simulink model "RBNN_NNT_timing_of_learning_1layerRBNN32order"  (R2019a)
settings: Solver=FixedStepAuto  StartTime=0.0  StopTime=inf  FixedStep=0.000001  RelTol=1e-3
libraries: dspstat3 x6, dspxfrm3 x1
(part 1 of 3)
settings Model: NumberOfSteps=3200  Creator=vardhah  LastModifiedBy=vardhah
settings DataIOCC: ReturnWorkspaceOutputs=off
settings DebuggingCC: UnderSpecifiedDimensionMsg=warning  ArithmeticOperatorsInVariantConditions=warning

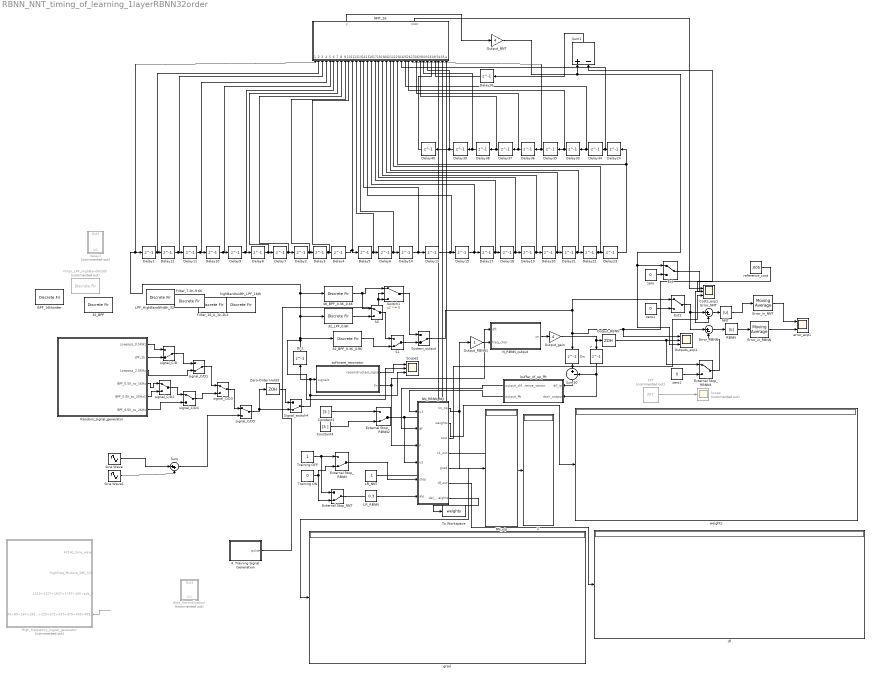
== system RBNN_NNT_timing_of_learning_1layerRBNN32order ==
  32_BPF : DiscreteFir  Tag=BlockMethodSubSystem  Coefficients=[0.0231270967292107159 0.0175343355945324977 0.00605221670125152041 0 0.00719679767045157404 0.0248456434051700405 0.0392205491332038511 0.0335684455675286375 -2.98876364449908766e-17 -0.0522852296501915767 -0.0987039819924426381 -0.111406686169706906 -0.0755372385277077452 1.2744675147390013e-17 0.0844207978699620387 0.139588301189413205 0.139588301189413205 0.0844207978699620387 1.2744675147390013e-17 -0.0755372385277077452 -0.111406686169706906 -0.0987039819924426381 -0.0522852296501915767 -2.98876364449908766e-17 0.0335684455675286375 0.0392205491332038511 0.0248456434051700405 0.00719679767045157404 0 0.00605221670125152041 0.0175343355945324977 0.0231270967292107159]  InputProcessing=Columns as channels (frame based)
  32_BPF_0.3K_0.9K : DiscreteFir  Tag=BlockMethodSubSystem  Coefficients=[0.00662659845422776134 0.00983298588902027475 0.00809664409693275702 -5.79647672595923754e-18 -0.0141669692502708264 -0.0321973902262055467 -0.0502752481995635894 -0.0637677476357453449 -0.0683320878931848175 -0.0610667384383032988 -0.0414056635152443217 -0.0115027859073064606 0.0240263013390189448 0.0589774451458855986 0.0868579066741778927 0.102309229147061892 0.102309229147061892 0.0868579066741778927 0.0589774451458855986 0.0240263013390189448 -0.0115027859073064606 -0.0414056635152443217 -0.0610667384383032988 -0.0683320878931848175 -0.0637677476357453449 -0.0502752481995635894 -0.0321973902262055467 -0.0141669692502708264 -5.79647672595923754e-18 0.00809664409693275702 0.00983298588902027475 0.00662659845422776134]  InputProcessing=Columns as channels (frame based)  SampleTime=0.0001
  32_LPF_0.6K : DiscreteFir  Tag=BlockMethodSubSystem  Coefficients=[-0.00901248685369954346 -0.0166232313070880447 -0.02293849257176446 -0.0268238277900753851 -0.0272765662653831481 -0.0235546351369226477 -0.0152840059258895229 -0.00253072016398011397 0.0141728632030948976 0.0338528489286080425 0.055168937477022735 0.0765332041207810732 0.0962604488743150494 0.112734006746784729 0.124568738621398098 0.130752918042798372 0.130752918042798372 0.124568738621398098 0.112734006746784729 0.0962604488743150494 0.0765332041207810732 0.055168937477022735 0.0338528489286080425 0.0141728632030948976 -0.00253072016398011397 -0.0152840059258895229 -0.0235546351369226477 -0.0272765662653831481 -0.0268238277900753851 -0.02293849257176446 -0.0166232313070880447 -0.00901248685369954346]  InputProcessing=Columns as channels (frame based)  SampleTime=0.0001
  4. Training Signal Generation : MATLAB Function  TreatAsAtomicUnit=on
  48_BPF_0.3K_0.6K : DiscreteFir  Tag=BlockMethodSubSystem  Coefficients=[0.0173870629140374378 0.0207423482676672884 0.0225684944558904275 0.0223574555139875765 0.0197817601251017959 0.0147549785512151154 0.00746744065508679611 -0.001608996203153008 -0.0117498180199336073 -0.0220390277764995618 -0.0314572377427717528 -0.0389877339734026607 -0.0437289550833909607 -0.0450005271887067293 -0.0424302142891804998 -0.0360109004456410225 -0.0261198472327749086 -0.0134966227084623806 0.00081920313306374482 0.0155848141621206405 0.0294754638356683092 0.0412174342630990259 0.0497181612101459114 0.0541791579705657028 0.0541791579705657028 0.0497181612101459114 0.0412174342630990259 0.0294754638356683092 0.0155848141621206405 0.00081920313306374482 -0.0134966227084623806 -0.0261198472327749086 -0.0360109004456410225 -0.0424302142891804998 -0.0450005271887067293 -0.0437289550833909607 -0.0389877339734026607 -0.0314572377427717528 -0.0220390277764995618 -0.0117498180199336073 -0.001608996203153008 0.00746744065508679611 0.0147549785512151154 0.0197817601251017959 0.0223574555139875765 0.0225684944558904275 0.0207423482676672884 0.0173870629140374378]  InputProcessing=Columns as channels (frame based)  SampleTime=0.0001
  BPF_16thorder : DiscreteFir  Tag=BlockMethodSubSystem  Coefficients=[-0.0560788660629819163 -0.080220031928137342 -0.085169812197034192 -0.0616477005407154097 -0.0104987832754634518 0.0560691321297696263 0.118166811935027122 0.155549755804414214 0.155549755804414214 0.118166811935027122 0.0560691321297696263 -0.0104987832754634518 -0.0616477005407154097 -0.085169812197034192 -0.080220031928137342 -0.0560788660629819163]  InputProcessing=Columns as channels (frame based)  SampleTime=0.0001
  Constant1 : Constant  Value=[5 ]
  Constant4 : Constant  Value=[3 ]
  Costs_exp1 : Scope  NumInputPorts=3
  Delay{1..24,33..40} (32 alike) : Delay  DelayLength=1  InitialCondition=0
  Dn : Delay  DelayLength=1  InitialCondition=0
  Dn1 : Delay  DelayLength=1  InitialCondition=0
  Error_NNT : Sum  Inputs=|+-
  Error_RBNN : Sum  Inputs=|+-
  Error_in_NNT : dspstat3/Moving Average  Method=Sliding window  ForgettingFactorPort=off  SpecifyWindowLength=on  WindowLength=32  ForgettingFactor=0.9  SimulateUsing=Code generation
  Error_in_RBNN : dspstat3/Moving Average  Method=Sliding window  ForgettingFactorPort=off  SpecifyWindowLength=on  WindowLength=32  ForgettingFactor=0.9  SimulateUsing=Code generation
  Ext : ManualSwitch
  Ext1 : ManualSwitch
  External Stop_NNT : ManualSwitch  CurrentSetting=0
  External Stop_RBNN : ManualSwitch  CurrentSetting=0
  External Stop_RBNN2 : ManualSwitch  CurrentSetting=0
  External Stop_RBNN3 : ManualSwitch
  FFT : dspxfrm3/FFT  Commented=on  FFTImplementation=Auto  CompMethod=Table lookup  TableOpt=NEW  TableOptActive=Speed  BitRevOrder=off  Normalize=off  InheritFFTLength=off  FFTLength=16  WrapInput=on  roundingMode=Floor  overflowMode=off  firstCoeffDataTypeStr=Inherit: Same word length as input  firstCoeffLastDataTypeStr=Inherit: Same word length as input  outputMin=[]  outputMax=[]
  Filter_16_A_1k-2k2 : DiscreteFir  Tag=BlockMethodSubSystem  Coefficients=[-0.198889914644374777 0.0882189428518377339 0.0736891495871065116 0.0638368801789635787 0.0566372642221577294 0.0523172683654103132 0.0494565343907736044 0.048157521822162791 0.048157521822162791 0.0494565343907736044 0.0523172683654103132 0.0566372642221577294 0.0638368801789635787 0.0736891495871065116 0.0882189428518377339 -0.198889914644374777]  InputProcessing=Columns as channels (frame based)  SampleTime=0.0001
  "Filter_7.2K-9.6K " : DiscreteFir  Tag=BlockMethodSubSystem  Coefficients=[-0.0120785049852322399 -0.0942455273574688279 0.0101245004695954266 0.125460404555770566 0.034165372769331126 -0.1614987160724079 -0.0984930555982914957 0.150982315564688691 0.150982315564688691 -0.0984930555982914957 -0.1614987160724079 0.034165372769331126 0.125460404555770566 0.0101245004695954266 -0.0942455273574688279 -0.0120785049852322399]  InputProcessing=Columns as channels (frame based)  SampleTime=0.0001
  Filter_LPF_HighBandWidth : DiscreteFir  Tag=BlockMethodSubSystem  Commented=on  Coefficients=[0.00257561197553052117 0.0149226993015543988 -0.0126813197622564593 0.0131583623867790739 -0.0109438145213804211 0.00462377218068549256 0.00574880781840408916 -0.0188595701191665473 0.032156879848246514 -0.042054633169390801 0.0443249918452583783 -0.0343435917303160365 0.00670297923827019304 0.0478068572768818173 -0.160206703181909604 0.618531838092966302 0.618531838092966302 -0.160206703181909604 0.0478068572768818173 0.00670297923827019304 -0.0343435917303160365 0.0443249918452583783 -0.042054633169390801 0.032156879848246514 -0.0188595701191665473 0.00574880781840408916 0.00462377218068549256 -0.0109438145213804211 0.0131583623867790739 -0.0126813197622564593 0.0149226993015543988 0.00257561197553052117]  InputProcessing=Columns as channels (frame based)  SampleTime=0.0001
  HIgh_frequency_signal_generator : Subsystem  Commented=on
  LPF_HighBandWidth_32 : DiscreteFir  Tag=BlockMethodSubSystem  Coefficients=[0.00257561197553052117 0.0149226993015543988 -0.0126813197622564593 0.0131583623867790739 -0.0109438145213804211 0.00462377218068549256 0.00574880781840408916 -0.0188595701191665473 0.032156879848246514 -0.042054633169390801 0.0443249918452583783 -0.0343435917303160365 0.00670297923827019304 0.0478068572768818173 -0.160206703181909604 0.618531838092966302 0.618531838092966302 -0.160206703181909604 0.0478068572768818173 0.00670297923827019304 -0.0343435917303160365 0.0443249918452583783 -0.042054633169390801 0.032156879848246514 -0.0188595701191665473 0.00574880781840408916 0.00462377218068549256 -0.0109438145213804211 0.0131583623867790739 -0.0126813197622564593 0.0149226993015543988 0.00257561197553052117]  InputProcessing=Columns as channels (frame based)  SampleTime=0.0001
  LR_NNT : Constant  Value=.1
  LR_RBNN : Constant  Value=0.3
  NNT : Abs
  NNT_16 : MATLAB Function  TreatAsAtomicUnit=on  SystemSampleTime=0.0001
  NN_RBNN_NN : MATLAB Function  TreatAsAtomicUnit=on
  NN_o/p : Display
  N_RBNN_output : MATLAB Function  TreatAsAtomicUnit=on
  Output_NNT : Gain  Gain=4
  Output_RBNN : ZeroOrderHold  SampleTime=-1
  Output_RBNN1 : Gain
  Output_gain : Gain  Gain=4
  Outputs_exp1 : Scope  NumInputPorts=3
  RBNN : Abs
  Random_signal_generator : Subsystem
  S1 : ManualSwitch  CurrentSetting=0
  S3 : ManualSwitch
  Scope : Scope  Commented=on
  Scope2 : Scope  NumInputPorts=3
  Signal_switch4 : ManualSwitch  CurrentSetting=0
  Sine Wave : Sin  Frequency=1297  SampleTime=0.0001
  Sine Wave1 : Sin  Frequency=2031  SampleTime=0.0001
  Sum : Sum  Inputs=|++
  Sum1 : Sum  Inputs=+-
  Sum50 : Sum  Inputs=|+-
  Switch1 : Switch  Criteria=u2 ~= 0
  "System_output " : ManualSwitch  CurrentSetting=0
  To Workspace : ToWorkspace  VariableName=weights  SaveFormat=Timeseries  SampleTime=-1
  Training OFF : Constant
  Training ON : Constant  Value=0
  Z : Display
  Zero-Order Hold3 : ZeroOrderHold  SampleTime=0.0001
  buffer_of_op_fft : MATLAB Function  TreatAsAtomicUnit=on
  data_Normalization : Subsystem  Commented=on
  delay1 : Subsystem  Commented=on
  df : Display
  error_exp1 : Scope  NumInputPorts=2
  grad : Display
  highBandwidth_LPF_16th : DiscreteFir  Tag=BlockMethodSubSystem  Coefficients=[-0.0297618438739734592 -0.0348768570143923456 0.0417652636536197108 0.0516071256815222451 -0.0669316025800295866 -0.0943151588376726635 0.157872597041064711 0.474640475929861472 0.474640475929861472 0.157872597041064711 -0.0943151588376726635 -0.0669316025800295866 0.0516071256815222451 0.0417652636536197108 -0.0348768570143923456 -0.0297618438739734592]  InputProcessing=Columns as channels (frame based)  SampleTime=0.0001
  reference_cost : Constant  Value=.005
  signal_C/D : ManualSwitch  CurrentSetting=0
  signal_C/D1 : ManualSwitch  CurrentSetting=0
  signal_C/D{2..5} (4 alike) : ManualSwitch
  software_rezonator : MATLAB Function  TreatAsAtomicUnit=on  SystemSampleTime=0.0001
  weights : Display
  y : Delay  DelayLength=1  InitialCondition=0
  zero : Constant  Value=0
  zero1 : Constant  Value=0
  "zero1 " : Constant  Value=0
  wires:
  software_rezonator/1(reconstructed_signal) -> Scope2/1
  software_rezonator/2(Fn) -> NN_RBNN_NN/3(F), N_RBNN_output/1(dft)
  N_RBNN_output/1(yn) -> Output_gain/1
  Dn/1 -> Sum50/1
  y/1 -> buffer_of_op_fft/2(rbnn_output), Sum50/2
  NN_RBNN_NN/1(nn_op) -> NN_o/p/1, Output_RBNN1/1
  Training OFF/1 -> External Stop_NNT/1, External Stop_RBNN/1
  Training ON/1 -> External Stop_NNT/2, External Stop_RBNN/2
  NN_RBNN_NN/3(cost) -> Costs_exp1/3
  NN_RBNN_NN/2(weights) -> weights/1
  NN_RBNN_NN/4(z1_out) -> Z/1
  Sum50/1 -> buffer_of_op_fft/1(dif_ip)
  buffer_of_op_fft/1(output_difference_vector) -> NN_RBNN_NN/2(df)
  buffer_of_op_fft/2(output_fft) -> NN_RBNN_NN/1(u1)
  NNT_16/1(y) -> Output_NNT/1
  Delay16/1 -> NNT_16/33(df)
  Delay4/1 -> NNT_16/11(X10), Delay5/1
  Delay6/1 -> Delay14/1, NNT_16/13(X12)
  Delay5/1 -> Delay6/1, NNT_16/12(X11)
  Delay2/1 -> Delay3/1, NNT_16/9(X8)
  Delay13/1 -> NNT_16/15(X14), Delay15/1
  Delay14/1 -> Delay13/1, NNT_16/14(X13)
  Delay10/1 -> NNT_16/5(X4), Delay9/1
  signal_C/D5/1 -> Zero-Order Hold3/1, Signal_switch4/2
  Delay3/1 -> NNT_16/10(X9), Delay4/1
  Delay7/1 -> Delay2/1, NNT_16/8(X7)
  Delay8/1 -> NNT_16/7(X6), Delay7/1
  Delay1/1 -> Delay12/1, NNT_16/2(X1)
  Delay9/1 -> NNT_16/6(X5), Delay8/1
  Delay12/1 -> NNT_16/3(X2), Delay11/1
  Delay11/1 -> NNT_16/4(X3), Delay10/1
  Sum1/1 -> Delay16/1
  Error_RBNN/1 -> RBNN/1
  Error_NNT/1 -> NNT/1
  LR_RBNN/1 -> NN_RBNN_NN/6(alp)
  RBNN/1 -> Error_in_RBNN/1
  NNT/1 -> Error_in_NNT/1
  Error_in_NNT/1 -> error_exp1/1
  Error_in_RBNN/1 -> error_exp1/2
  External Stop_NNT/1 -> NNT_16/34(stop)
  Output_gain/1 -> y/1, Output_RBNN/1
  LR_NNT/1 -> NNT_16/35(alpha_l)
  HIgh_frequency_signal_generator/4(43+89+167+193+229+271+337+379+409+499_H) -> ?
  Zero-Order Hold3/1 -> Signal_switch4/1
  FFT/1 -> Scope/1
  Switch1/1 -> "System_output "/1
  Constant1/1 -> External Stop_RBNN2/1
  4. Training Signal Generation/1(pulse) -> Switch1/3, Switch1/2
  Constant4/1 -> External Stop_RBNN2/2
  External Stop_RBNN2/1 -> NNT_16/36(a), NN_RBNN_NN/4(u2)
  Output_NNT/1 -> Outputs_exp1/3, Ext/1, Sum1/1
  S3/1 -> S1/1
  S1/1 -> "System_output "/2
  Output_RBNN1/1 -> N_RBNN_output/2(freq_char)
  NN_RBNN_NN/5(grad) -> grad/1
  Output_RBNN/1 -> External Stop_RBNN3/1, Outputs_exp1/2
  NN_RBNN_NN/6(df_out) -> df/1
  "System_output "/1 -> Ext1/1, Dn/1, Sum1/2, Outputs_exp1/1
  NN_RBNN_NN/7(del_weights) -> To Workspace/1
  Signal_switch4/1 -> Scope2/3, Dn1/1, software_rezonator/1(signalz)
  signal_C/D/1 -> signal_C/D1/1
  Random_signal_generator/3(Lowpass_2.5KHz) -> signal_C/D1/2
  Random_signal_generator/4(BPF_0.5K_to_1KHz) -> signal_C/D2/1
  signal_C/D3/1 -> signal_C/D5/1
  signal_C/D1/1 -> signal_C/D3/1
  Random_signal_generator/1(Lowpass_0.5KHz) -> signal_C/D/1
  Random_signal_generator/2(LPF_1k) -> signal_C/D/2
  "zero1 "/1 -> External Stop_RBNN3/2
  External Stop_RBNN3/1 -> Error_RBNN/2
  Ext/1 -> Error_NNT/2
  zero/1 -> Ext/2
  zero1/1 -> Ext1/2
  Ext1/1 -> Error_RBNN/1, Error_NNT/1
  reference_cost/1 -> Costs_exp1/2
  Random_signal_generator/5(BPF_0.5K_to_2KHz1) -> signal_C/D2/2
  signal_C/D2/1 -> signal_C/D4/1
  Random_signal_generator/6(BPF_0.5K_to_2KHz) -> signal_C/D4/2
  signal_C/D4/1 -> signal_C/D3/2
  External Stop_RBNN/1 -> NN_RBNN_NN/5(stop)
  Sine Wave/1 -> Sum/1
  Sine Wave1/1 -> Sum/2
  Sum/1 -> signal_C/D5/2
  Delay15/1 -> Delay17/1, NNT_16/16(X15)
  Delay17/1 -> NNT_16/17(X16), Delay18/1
  Delay18/1 -> NNT_16/18(X17), Delay19/1
  Delay19/1 -> NNT_16/19(X18), Delay20/1
  Delay20/1 -> NNT_16/20(X19), Delay21/1
  Delay21/1 -> NNT_16/21(X20), Delay22/1
  Delay22/1 -> NNT_16/22(X21), Delay23/1
  Delay23/1 -> NNT_16/23(X22), Delay24/1
  Delay24/1 -> Delay34/1, NNT_16/24(X23)
  Delay34/1 -> Delay33/1, NNT_16/25(X24)
  Delay33/1 -> Delay35/1, NNT_16/26(X25)
  Delay35/1 -> Delay36/1, NNT_16/27(X26)
  Delay36/1 -> Delay37/1, NNT_16/28(X27)
  Delay37/1 -> Delay38/1, NNT_16/29(X28)
  Delay38/1 -> Delay39/1, NNT_16/30(X29)
  Delay39/1 -> NNT_16/31(X30), Delay40/1
  Delay40/1 -> NNT_16/32(X31)
  NNT_16/2(cost) -> Costs_exp1/1
  32_BPF_0.3K_0.9K/1 -> S1/2
  48_BPF_0.3K_0.6K/1 -> S3/1, Switch1/1
  32_LPF_0.6K/1 -> S3/2
  Dn1/1 -> 32_BPF_0.3K_0.9K/1, 32_LPF_0.6K/1, 48_BPF_0.3K_0.6K/1, Delay1/1, NNT_16/1(X0), Scope2/2

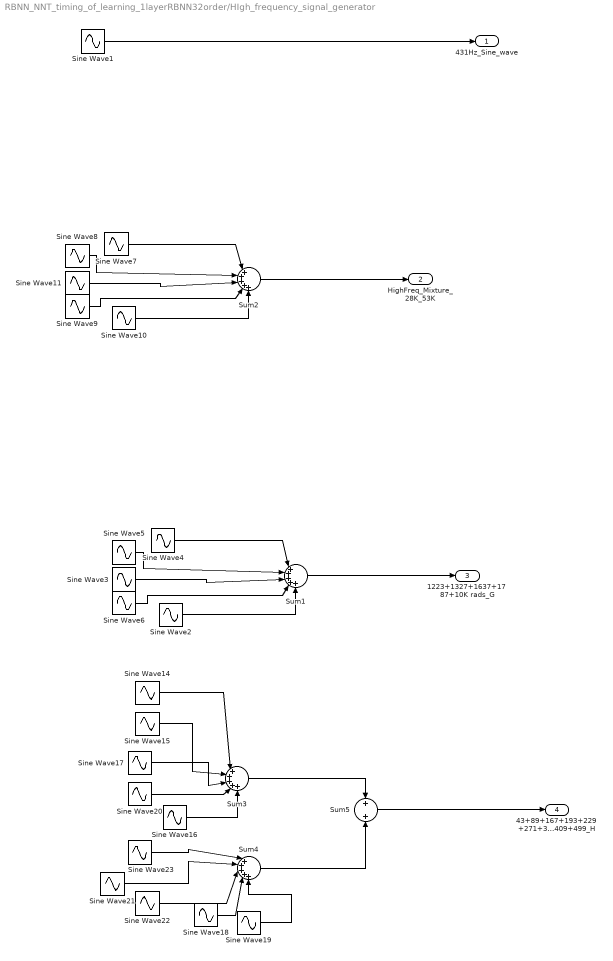
== system RBNN_NNT_timing_of_learning_1layerRBNN32order/HIgh_frequency_signal_generator ==
  Sine Wave1 : Sin  Amplitude=0.5  Frequency=23000  SampleTime=0.0001
  Sine Wave10 : Sin  Amplitude=0.5  Frequency=7000  SampleTime=0
  Sine Wave11 : Sin  Amplitude=2  Frequency=3637  SampleTime=0
  Sine Wave14 : Sin  Amplitude=0.1  Frequency=43  SampleTime=0
  Sine Wave15 : Sin  Amplitude=0.1  Frequency=89  SampleTime=0
  Sine Wave16 : Sin  Amplitude=0.1  Frequency=229  SampleTime=0
  Sine Wave17 : Sin  Amplitude=0.1  Frequency=167  SampleTime=0
  Sine Wave18 : Sin  Amplitude=0.1  Frequency=409  SampleTime=0
  Sine Wave19 : Sin  Amplitude=0.1  Frequency=499  SampleTime=0
  Sine Wave2 : Sin  Amplitude=0  Frequency=5000  SampleTime=0
  Sine Wave20 : Sin  Amplitude=0.1  Frequency=193  SampleTime=0
  Sine Wave21 : Sin  Amplitude=0.1  Frequency=337  SampleTime=0
  Sine Wave22 : Sin  Amplitude=0.1  Frequency=379  SampleTime=0
  Sine Wave23 : Sin  Amplitude=0.1  Frequency=271  SampleTime=0
  Sine Wave3 : Sin  Amplitude=0.25  Frequency=200  SampleTime=0
  Sine Wave4 : Sin  Amplitude=0.25  Frequency=50  SampleTime=0
  Sine Wave5 : Sin  Amplitude=0.25  Frequency=100  SampleTime=0
  Sine Wave6 : Sin  Amplitude=0.25  Frequency=1787  SampleTime=0
  Sine Wave7 : Sin  Amplitude=2  Frequency=2230  SampleTime=0
  Sine Wave8 : Sin  Amplitude=2  Frequency=5927  SampleTime=0
  Sine Wave9 : Sin  Amplitude=2  Frequency=3787  SampleTime=0
  Sum{1..4} (4 alike) : Sum  Inputs=|+++++
  Sum5 : Sum
  431Hz_Sine_wave : Outport
  HighFreq_Mixture_28K_53K : Outport  Port=2
  1223+1327+1637+1787+10K rads_G : Outport  Port=3
  43+89+167+193+229+271+337+379+409+499_H : Outport  Port=4
  wires:
  Sine Wave9/1 -> Sum2/4
  Sine Wave7/1 -> Sum2/1
  Sine Wave10/1 -> Sum2/5
  Sine Wave8/1 -> Sum2/2
  Sine Wave11/1 -> Sum2/3
  Sum2/1 -> HighFreq_Mixture_28K_53K/1
  Sine Wave23/1 -> Sum4/1
  Sine Wave17/1 -> Sum3/3
  Sine Wave22/1 -> Sum4/3
  Sine Wave18/1 -> Sum4/4
  Sine Wave19/1 -> Sum4/5
  Sine Wave5/1 -> Sum1/2
  Sine Wave20/1 -> Sum3/4
  Sine Wave4/1 -> Sum1/1
  Sine Wave14/1 -> Sum3/1
  Sine Wave15/1 -> Sum3/2
  Sine Wave21/1 -> Sum4/2
  Sine Wave16/1 -> Sum3/5
  Sine Wave6/1 -> Sum1/4
  Sum4/1 -> Sum5/2
  Sum3/1 -> Sum5/1
  Sine Wave2/1 -> Sum1/5
  Sine Wave3/1 -> Sum1/3
  Sum1/1 -> 1223+1327+1637+1787+10K rads_G/1
  Sum5/1 -> 43+89+167+193+229+271+337+379+409+499_H/1
  Sine Wave1/1 -> 431Hz_Sine_wave/1
